simulink model "ForceControl_Quadruped_vmc"  (R2018b)
settings: Solver=FixedStepAuto  StartTime=0.0  StopTime=2  FixedStep=0.001  RelTol=1e-3  EnableMultiTasking=on
undefined symbols (not defined in the file or in its folder): robot, X, Y, Z
libraries: sm_lib x43, nesl_utility x32, Contact_Forces_Lib x4
(part 3 of 3)

== matlab function ForceControl_Quadruped_vmc/controller/inverse kinematics3 ==
  data: x input; y input; z input; shoulder output; hip output; knee output
function [shoulder,hip,knee]= coord2theta(x,y,z)
% L1=75.0;
% L2=415.0;
% L3=408.0;


% temp = (L1*L1+L2*L2-x*x-z*z)/(2*L1*L2);
% if temp>1
%     temp = 1;
% elseif temp<-1
%     temp=1;
% end
% theta2 = pi-acos(temp);
% 
% temp = (x*x+z*z+L1*L1-L2*L2)/(2*sqrt(x*x+z*z)*L1);
% if temp>1
%     temp = 1;
% elseif temp<-1
%     temp=1;
% end
% if(x>0)
%     theta1 = abs(atan(x/z))-acos(temp);
% elseif(x<0)
%     theta1 = -abs(atan(x/z))-acos(temp);
% else
%     theta1 = -acos(temp);

L1=0;
L2=0.4;
L3=0.4;

shoulder=atan(-y/z);

%髋关节到足端长度的平方
L_H2E_2=x*x+(y-L1*sin(shoulder))*(y-L1*sin(shoulder))+(z+L1*cos(shoulder))*(z+L1*cos(shoulder));
%髋关节到足端长度
L_H2E=sqrt(L_H2E_2);

temp = (L2*L2+L_H2E_2-L3*L3)/(2*L_H2E*L2);
if temp>1
    temp = 1;
elseif temp<-1
    temp = -1;
end
Zeta=acos(temp);
hip=atan(x/(sqrt(y*y+z*z)-L1))-Zeta;

temp = (L2*L2+L3*L3-L_H2E_2)/(2*L2*L3);
if temp>1
    temp = 1;
elseif temp<-1
    temp = -1;
end
knee=pi-acos(temp);

== matlab function ForceControl_Quadruped_vmc/controller/inverse kinematics4 ==
  data: x input; y input; z input; shoulder output; hip output; knee output
function [shoulder,hip,knee]= coord2theta(x,y,z)
% L1=75.0;
% L2=415.0;
% L3=408.0;


% temp = (L1*L1+L2*L2-x*x-z*z)/(2*L1*L2);
% if temp>1
%     temp = 1;
% elseif temp<-1
%     temp=1;
% end
% theta2 = pi-acos(temp);
% 
% temp = (x*x+z*z+L1*L1-L2*L2)/(2*sqrt(x*x+z*z)*L1);
% if temp>1
%     temp = 1;
% elseif temp<-1
%     temp=1;
% end
% if(x>0)
%     theta1 = abs(atan(x/z))-acos(temp);
% elseif(x<0)
%     theta1 = -abs(atan(x/z))-acos(temp);
% else
%     theta1 = -acos(temp);

L1=0;
L2=0.4;
L3=0.4;

shoulder=atan(-y/z);

%髋关节到足端长度的平方
L_H2E_2=x*x+(y-L1*sin(shoulder))*(y-L1*sin(shoulder))+(z+L1*cos(shoulder))*(z+L1*cos(shoulder));
%髋关节到足端长度
L_H2E=sqrt(L_H2E_2);

temp = (L2*L2+L_H2E_2-L3*L3)/(2*L_H2E*L2);
if temp>1
    temp = 1;
elseif temp<-1
    temp = -1;
end
Zeta=acos(temp);
hip=atan(x/(sqrt(y*y+z*z)-L1))-Zeta;

temp = (L2*L2+L3*L3-L_H2E_2)/(2*L2*L3);
if temp>1
    temp = 1;
elseif temp<-1
    temp = -1;
end
knee=pi-acos(temp);

== matlab function ForceControl_Quadruped_vmc/controller/trajectory generate1 ==
  data: timer1 input; first_run input; timer1 output; first_run output; LegFL output; LegFR output; LegRR output; LegRL output; run input; roll_angle input; pitch_angle input; yaw_angle input; Body_x input; Body_y input; Body_z input
function [timer1,first_run,LegFL,LegFR,LegRR,LegRL] = gesture( timer1,first_run,run,roll_angle,pitch_angle,yaw_angle,Body_x,Body_y,Body_z)
Ts = 0.75;

if run
    timer1 = timer1+0.001;
    if timer1>=Ts
        timer1 = 0;
    end
end

Xs = -0.1;
Xe = 0.1;

Ys = 0;

Zs = -0.55;
H = 0.15;

body_len_half = 0.35;
body_width_half = 0.2;

Body2FL = [body_len_half,body_width_half,0]';
Body2FR = [body_len_half,-body_width_half,0]';
Body2RR = [-body_len_half,-body_width_half,0]';
Body2RL = [-body_len_half,body_width_half,0]';

Body2FL_trans = [eye(3,3),Body2FL;
    zeros(1,3),1];
Body2FR_trans = [eye(3,3),Body2FR;
    zeros(1,3),1];
Body2RR_trans = [eye(3,3),Body2RR;
    zeros(1,3),1];
Body2RL_trans = [eye(3,3),Body2RL;
    zeros(1,3),1];

roll = roll_angle*pi/180;  
pitch = pitch_angle*pi/180; 
yaw = yaw_angle*pi/180;    

R_roll=[1,0,0,0;
        0,cos(roll),-sin(roll),0;
        0,sin(roll),cos(roll),0;
        0,0,0,1];

R_pitch=[cos(pitch),0,sin(pitch),0;
        0,1,0,0;
        -sin(pitch),0,cos(pitch),0;
        0,0,0,1];

R_yaw=[cos(yaw),-sin(yaw),0,0;
        sin(yaw),cos(yaw),0,0;
        0,0,1,0;
        0,0,0,1];

Body_Trans=[eye(3,3),[Body_x,Body_y,Body_z]';
            zeros(1,3),1];

if first_run
    if timer1>0 && timer1<=0.5*Ts 
        sigma = 2*pi*(timer1)/(0.5*Ts);
        x_f = (Xe-Xs)*((sigma-sin(sigma))/(2*pi))+Xs;  
        x_b = (Xs-Xe)*((sigma-sin(sigma))/(2*pi))+Xe;  
        z_up = H*(1-cos(sigma))/2+Zs;
        
        LegFL = [Xs,-Ys,Zs]';
        LegFR = [x_f,Ys,z_up]';
        LegRR = [Xs,Ys,Zs]';
        LegRL = [x_f,-Ys,z_up]';
    else
        LegFL = [Xs,-Ys,Zs]';
        LegFR = [Xs,Ys,Zs]';
        LegRR = [Xs,Ys,Zs]';
        LegRL = [Xs,-Ys,Zs]';
    end
    if timer1>0.5*Ts
        timer1 = 0;
        first_run = 0;
    end
else
    if timer1>0 && timer1<=0.5*Ts 
        sigma = 2*pi*(timer1)/(0.5*Ts);
        x_f = (Xe-Xs)*((sigma-sin(sigma))/(2*pi))+Xs;  
        x_b = (Xs-Xe)*((sigma-sin(sigma))/(2*pi))+Xe;  
        z_up = H*(1-cos(sigma))/2+Zs; 
        
        O_FL = [body_len_half+x_f,body_width_half,z_up,1]';
        O_FR = [body_len_half+x_b,-body_width_half,Zs,1]';
        O_RR = [-body_len_half+x_f,-body_width_half,z_up,1]';
        O_RL = [-body_len_half+x_b,body_width_half,Zs,1]';
        
    elseif timer1>0.5*Ts && timer1<Ts 
        sigma = 2*pi*(timer1-0.5*Ts)/(0.5*Ts);
        x_f = (Xe-Xs)*((sigma-sin(sigma))/(2*pi))+Xs;
        x_b = (Xs-Xe)*((sigma-sin(sigma))/(2*pi))+Xe;  
        z_up = H*(1-cos(sigma))/2+Zs;
              
        O_FL = [body_len_half+x_b,body_width_half,Zs,1]';
        O_FR = [body_len_half+x_f,-body_width_half,z_up,1]';
        O_RR = [-body_len_half+x_b,-body_width_half,Zs,1]';
        O_RL = [-body_len_half+x_f,body_width_half,z_up,1]';
    else 
        roll = 0;
        pitch = 0;
        yaw = 0;
        Body_x = 0;
        Body_y = 0;
        Body_z = 0;
        
        R_roll=[1,0,0,0;
                0,cos(roll),-sin(roll),0;
                0,sin(roll),cos(roll),0;
                0,0,0,1];
        R_pitch=[cos(pitch),0,sin(pitch),0;
                0,1,0,0;
                -sin(pitch),0,cos(pitch),0;
                0,0,0,1];
        R_yaw=[cos(yaw),-sin(yaw),0,0;
                sin(yaw),cos(yaw),0,0;
                0,0,1,0;
                0,0,0,1];
        Body_Trans=[eye(3,3),[Body_x,Body_y,Body_z]';
                    zeros(1,3),1];
        O_FL = [body_len_half+Xs,body_width_half-Ys,Zs,1]';
        O_FR = [body_len_half+Xs,-body_width_half+Ys,Zs,1]';
        O_RR = [-body_len_half+Xs,-body_width_half+Ys,Zs,1]';
        O_RL = [-body_len_half+Xs,body_width_half-Ys,Zs,1]';
    end
    P_FL = inv(Body2FL_trans)*R_roll*R_pitch*R_yaw*Body_Trans*O_FL;
    P_FR = inv(Body2FR_trans)*R_roll*R_pitch*R_yaw*Body_Trans*O_FR;
    P_RR = inv(Body2RR_trans)*R_roll*R_pitch*R_yaw*Body_Trans*O_RR;
    P_RL = inv(Body2RL_trans)*R_roll*R_pitch*R_yaw*Body_Trans*O_RL;

    LegFL = P_FL(1:3);
    LegFR = P_FR(1:3);
    LegRR = P_RR(1:3);
    LegRL = P_RL(1:3);
end

== matlab function ForceControl_Quadruped_vmc/controller/inverse kinematics2 ==
  data: x input; y input; z input; shoulder output; hip output; knee output
function [shoulder,hip,knee]= coord2theta(x,y,z)
% L1=75.0;
% L2=415.0;
% L3=408.0;


% temp = (L1*L1+L2*L2-x*x-z*z)/(2*L1*L2);
% if temp>1
%     temp = 1;
% elseif temp<-1
%     temp=1;
% end
% theta2 = pi-acos(temp);
% 
% temp = (x*x+z*z+L1*L1-L2*L2)/(2*sqrt(x*x+z*z)*L1);
% if temp>1
%     temp = 1;
% elseif temp<-1
%     temp=1;
% end
% if(x>0)
%     theta1 = abs(atan(x/z))-acos(temp);
% elseif(x<0)
%     theta1 = -abs(atan(x/z))-acos(temp);
% else
%     theta1 = -acos(temp);

L1=0;
L2=0.4;
L3=0.4;

shoulder=atan(-y/z);

%髋关节到足端长度的平方
L_H2E_2=x*x+(y-L1*sin(shoulder))*(y-L1*sin(shoulder))+(z+L1*cos(shoulder))*(z+L1*cos(shoulder));
%髋关节到足端长度
L_H2E=sqrt(L_H2E_2);

temp = (L2*L2+L_H2E_2-L3*L3)/(2*L_H2E*L2);
if temp>1
    temp = 1;
elseif temp<-1
    temp = -1;
end
Zeta=acos(temp);
hip=atan(x/(sqrt(y*y+z*z)-L1))-Zeta;

temp = (L2*L2+L3*L3-L_H2E_2)/(2*L2*L3);
if temp>1
    temp = 1;
elseif temp<-1
    temp = -1;
end
knee=pi-acos(temp);

== matlab function ForceControl_Quadruped_vmc/FL/MATLAB Function1 ==
  data: q input; coord output
function coord = forward_kinematics(q)

%肩关节中心为坐标原点
%坐标轴满足右手定则，x轴朝右，z轴朝上，逆时针为旋转正方向

%L0(shoulder length) L1(upper leg length) L2(lower leg length)
%theta0(shoulder angle) theta1(hip angle) theta2(knee angle)

%     x = L1*sin(theta1)+L2*sin(theta1+theta2);
%     y = sin(theta0)*(L1*cos(theta1)+L2*cos(theta1+theta2));
%     z = -cos(theta0)*(L1*cos(theta1)+L2*cos(theta1+theta2));

theta0 = q(1);
theta1 = q(2);
theta2 = q(3);

L0 = 0;
L1 = 0.4;
L2 = 0.4;

s0 = sin(theta0);s1 = sin(theta1);s2 = sin(theta2);
c0 = cos(theta0);c1 = cos(theta1);c2 = cos(theta2);
s12 = sin(theta1+theta2);c12 = cos(theta1+theta2);

x = L1*s1+L2*s12;
y = s0*(L1*c1+L2*c12);
z = -c0*(L1*c1+L2*c12);

coord = [x,y,z];

== matlab function ForceControl_Quadruped_vmc/FL/MATLAB Function2 ==
  data: pos input; vel output; pos_last input; pos output; first_run input; first_run output
function [vel,pos,first_run] = Pos2Vel(pos,pos_last,first_run)

if first_run
    x_pos_last = pos(1);
    y_pos_last = pos(2);
    z_pos_last = pos(3);
    first_run = 0;
else
    x_pos_last = pos_last(1);
    y_pos_last = pos_last(2);
    z_pos_last = pos_last(3);
end

x_pos = pos(1);
y_pos = pos(2);
z_pos = pos(3);

x_vel = (x_pos-x_pos_last)/0.001;
y_vel = (y_pos-y_pos_last)/0.001;
z_vel = (z_pos-z_pos_last)/0.001;

vel = [x_vel,y_vel,z_vel];

== matlab function ForceControl_Quadruped_vmc/FL/MATLAB Function ==
  data: fx input; tau0 output; fy input; fz input; tau1 output; tau2 output; theta input
function [tau0,tau1,tau2] = fcn(fx,fy,fz,theta)
L0 = 0;
L1 = 0.4;
L2 = 0.4;

theta0 = theta(1);theta1 = theta(2);theta2 = theta(3);
s0 = sin(theta0);s1 = sin(theta1);s2 = sin(theta2);
c0 = cos(theta0);c1 = cos(theta1);c2 = cos(theta2);
s12 = sin(theta1+theta2);c12 = cos(theta1+theta2);

% x = L1*s1+L2*s12;
% y = s0*(L1*c1+L2*c12);
% z = -c0*(L1*c1+L2*c12);


J = [0 L1*c1+L2*c12 L2*c12;
    c0*(L1*c1+L2*c12) -s0*(L1*s1+L2*s12) -s0*(L2*s12);
    s0*(L1*c1+L2*c12) c0*(L1*s1+L2*s12) c0*(L2*s12)];

F = [fx;fy;fz];
tau = J'*F;

tau0 = tau(1);
tau1 = tau(2);
tau2 = tau(3);

== matlab function ForceControl_Quadruped_vmc/FL1/MATLAB Function ==
  data: fx input; tau0 output; fy input; fz input; tau1 output; tau2 output; theta input
function [tau0,tau1,tau2] = fcn(fx,fy,fz,theta)
L0 = 0;
L1 = 0.4;
L2 = 0.4;

theta0 = theta(1);theta1 = theta(2);theta2 = theta(3);
s0 = sin(theta0);s1 = sin(theta1);s2 = sin(theta2);
c0 = cos(theta0);c1 = cos(theta1);c2 = cos(theta2);
s12 = sin(theta1+theta2);c12 = cos(theta1+theta2);

% x = L1*s1+L2*s12;
% y = s0*(L1*c1+L2*c12);
% z = -c0*(L1*c1+L2*c12);


J = [0 L1*c1+L2*c12 L2*c12;
    c0*(L1*c1+L2*c12) -s0*(L1*s1+L2*s12) -s0*(L2*s12);
    s0*(L1*c1+L2*c12) c0*(L1*s1+L2*s12) c0*(L2*s12)];

F = [fx;fy;fz];
tau = J'*F;

tau0 = tau(1);
tau1 = tau(2);
tau2 = tau(3);

== matlab function ForceControl_Quadruped_vmc/FL1/MATLAB Function1 ==
  data: q input; coord output
function coord = forward_kinematics(q)

%肩关节中心为坐标原点
%坐标轴满足右手定则，x轴朝右，z轴朝上，逆时针为旋转正方向

%L0(shoulder length) L1(upper leg length) L2(lower leg length)
%theta0(shoulder angle) theta1(hip angle) theta2(knee angle)

%     x = L1*sin(theta1)+L2*sin(theta1+theta2);
%     y = sin(theta0)*(L1*cos(theta1)+L2*cos(theta1+theta2));
%     z = -cos(theta0)*(L1*cos(theta1)+L2*cos(theta1+theta2));

theta0 = q(1);
theta1 = q(2);
theta2 = q(3);

L0 = 0;
L1 = 0.4;
L2 = 0.4;

s0 = sin(theta0);s1 = sin(theta1);s2 = sin(theta2);
c0 = cos(theta0);c1 = cos(theta1);c2 = cos(theta2);
s12 = sin(theta1+theta2);c12 = cos(theta1+theta2);

x = L1*s1+L2*s12;
y = s0*(L1*c1+L2*c12);
z = -c0*(L1*c1+L2*c12);

coord = [x,y,z];

== matlab function ForceControl_Quadruped_vmc/FL1/MATLAB Function2 ==
  data: pos input; vel output; pos_last input; pos output; first_run input; first_run output
function [vel,pos,first_run] = Pos2Vel(pos,pos_last,first_run)

if first_run
    x_pos_last = pos(1);
    y_pos_last = pos(2);
    z_pos_last = pos(3);
    first_run = 0;
else
    x_pos_last = pos_last(1);
    y_pos_last = pos_last(2);
    z_pos_last = pos_last(3);
end

x_pos = pos(1);
y_pos = pos(2);
z_pos = pos(3);

x_vel = (x_pos-x_pos_last)/0.001;
y_vel = (y_pos-y_pos_last)/0.001;
z_vel = (z_pos-z_pos_last)/0.001;

vel = [x_vel,y_vel,z_vel];

== matlab function ForceControl_Quadruped_vmc/FL2/MATLAB Function ==
  data: fx input; tau0 output; fy input; fz input; tau1 output; tau2 output; theta input
function [tau0,tau1,tau2] = fcn(fx,fy,fz,theta)
L0 = 0;
L1 = 0.4;
L2 = 0.4;

theta0 = theta(1);theta1 = theta(2);theta2 = theta(3);
s0 = sin(theta0);s1 = sin(theta1);s2 = sin(theta2);
c0 = cos(theta0);c1 = cos(theta1);c2 = cos(theta2);
s12 = sin(theta1+theta2);c12 = cos(theta1+theta2);

% x = L1*s1+L2*s12;
% y = s0*(L1*c1+L2*c12);
% z = -c0*(L1*c1+L2*c12);


J = [0 L1*c1+L2*c12 L2*c12;
    c0*(L1*c1+L2*c12) -s0*(L1*s1+L2*s12) -s0*(L2*s12);
    s0*(L1*c1+L2*c12) c0*(L1*s1+L2*s12) c0*(L2*s12)];

F = [fx;fy;fz];
tau = J'*F;

tau0 = tau(1);
tau1 = tau(2);
tau2 = tau(3);

== matlab function ForceControl_Quadruped_vmc/FL2/MATLAB Function1 ==
  data: q input; coord output
function coord = forward_kinematics(q)

%肩关节中心为坐标原点
%坐标轴满足右手定则，x轴朝右，z轴朝上，逆时针为旋转正方向

%L0(shoulder length) L1(upper leg length) L2(lower leg length)
%theta0(shoulder angle) theta1(hip angle) theta2(knee angle)

%     x = L1*sin(theta1)+L2*sin(theta1+theta2);
%     y = sin(theta0)*(L1*cos(theta1)+L2*cos(theta1+theta2));
%     z = -cos(theta0)*(L1*cos(theta1)+L2*cos(theta1+theta2));

theta0 = q(1);
theta1 = q(2);
theta2 = q(3);

L0 = 0;
L1 = 0.4;
L2 = 0.4;

s0 = sin(theta0);s1 = sin(theta1);s2 = sin(theta2);
c0 = cos(theta0);c1 = cos(theta1);c2 = cos(theta2);
s12 = sin(theta1+theta2);c12 = cos(theta1+theta2);

x = L1*s1+L2*s12;
y = s0*(L1*c1+L2*c12);
z = -c0*(L1*c1+L2*c12);

coord = [x,y,z];

== matlab function ForceControl_Quadruped_vmc/FL2/MATLAB Function2 ==
  data: pos input; vel output; pos_last input; pos output; first_run input; first_run output
function [vel,pos,first_run] = Pos2Vel(pos,pos_last,first_run)

if first_run
    x_pos_last = pos(1);
    y_pos_last = pos(2);
    z_pos_last = pos(3);
    first_run = 0;
else
    x_pos_last = pos_last(1);
    y_pos_last = pos_last(2);
    z_pos_last = pos_last(3);
end

x_pos = pos(1);
y_pos = pos(2);
z_pos = pos(3);

x_vel = (x_pos-x_pos_last)/0.001;
y_vel = (y_pos-y_pos_last)/0.001;
z_vel = (z_pos-z_pos_last)/0.001;

vel = [x_vel,y_vel,z_vel];

== matlab function ForceControl_Quadruped_vmc/FL3/MATLAB Function ==
  data: fx input; tau0 output; fy input; fz input; tau1 output; tau2 output; theta input
function [tau0,tau1,tau2] = fcn(fx,fy,fz,theta)
L0 = 0;
L1 = 0.4;
L2 = 0.4;

theta0 = theta(1);theta1 = theta(2);theta2 = theta(3);
s0 = sin(theta0);s1 = sin(theta1);s2 = sin(theta2);
c0 = cos(theta0);c1 = cos(theta1);c2 = cos(theta2);
s12 = sin(theta1+theta2);c12 = cos(theta1+theta2);

% x = L1*s1+L2*s12;
% y = s0*(L1*c1+L2*c12);
% z = -c0*(L1*c1+L2*c12);


J = [0 L1*c1+L2*c12 L2*c12;
    c0*(L1*c1+L2*c12) -s0*(L1*s1+L2*s12) -s0*(L2*s12);
    s0*(L1*c1+L2*c12) c0*(L1*s1+L2*s12) c0*(L2*s12)];

F = [fx;fy;fz];
tau = J'*F;

tau0 = tau(1);
tau1 = tau(2);
tau2 = tau(3);

== matlab function ForceControl_Quadruped_vmc/FL3/MATLAB Function1 ==
  data: q input; coord output
function coord = forward_kinematics(q)

%肩关节中心为坐标原点
%坐标轴满足右手定则，x轴朝右，z轴朝上，逆时针为旋转正方向

%L0(shoulder length) L1(upper leg length) L2(lower leg length)
%theta0(shoulder angle) theta1(hip angle) theta2(knee angle)

%     x = L1*sin(theta1)+L2*sin(theta1+theta2);
%     y = sin(theta0)*(L1*cos(theta1)+L2*cos(theta1+theta2));
%     z = -cos(theta0)*(L1*cos(theta1)+L2*cos(theta1+theta2));

theta0 = q(1);
theta1 = q(2);
theta2 = q(3);

L0 = 0;
L1 = 0.4;
L2 = 0.4;

s0 = sin(theta0);s1 = sin(theta1);s2 = sin(theta2);
c0 = cos(theta0);c1 = cos(theta1);c2 = cos(theta2);
s12 = sin(theta1+theta2);c12 = cos(theta1+theta2);

x = L1*s1+L2*s12;
y = s0*(L1*c1+L2*c12);
z = -c0*(L1*c1+L2*c12);

coord = [x,y,z];

== matlab function ForceControl_Quadruped_vmc/FL3/MATLAB Function2 ==
  data: pos input; vel output; pos_last input; pos output; first_run input; first_run output
function [vel,pos,first_run] = Pos2Vel(pos,pos_last,first_run)

if first_run
    x_pos_last = pos(1);
    y_pos_last = pos(2);
    z_pos_last = pos(3);
    first_run = 0;
else
    x_pos_last = pos_last(1);
    y_pos_last = pos_last(2);
    z_pos_last = pos_last(3);
end

x_pos = pos(1);
y_pos = pos(2);
z_pos = pos(3);

x_vel = (x_pos-x_pos_last)/0.001;
y_vel = (y_pos-y_pos_last)/0.001;
z_vel = (z_pos-z_pos_last)/0.001;

vel = [x_vel,y_vel,z_vel];

== matlab function ForceControl_Quadruped_vmc/controller1/MATLAB Function ==
  data: t input; theta_t output; theta_t_d output; theta_t_d2 output
function [theta_t,theta_t_d,theta_t_d2] = traj(t)

tf=2;
theta_0=0;
theta_f=pi/6;

a0=theta_0;
a1=0;
a2=3/(tf^2)*(theta_f-theta_0);
a3=-2/(tf^3)*(theta_f-theta_0);

theta_t=a0+a1.*t+a2.*t.^2+a3.*t.^3;
theta_t_d=a1+2*a2.*t+3*a3*t.^2;
theta_t_d2=2*a2+6*a3.*t;

== matlab function ForceControl_Quadruped_vmc/controller1/MATLAB Function1 ==
  data: theta input; theta_d input; q input; tau output; q_d input; q_d2 input
function tau  = dynamics(theta,theta_d,q,q_d,q_d2)
%DYNAMICS 此处显示有关此函数的摘要
%   此处显示详细说明
% I=1/12*m*(L1^2+L2^2) 
% 质量50KG，长宽高分别为0.8，0.4，0.2
% x轴，y轴，z轴分别平行于长宽高方向，原点建立在几何中心
mp = 50;

Ix=1/12*mp*(0.4^2+0.2^2);
Iy=1/12*mp*(0.8^2+0.2^2);
Iz=1/12*mp*(0.8^2+0.4^2);

theta_x=theta(1);theta_y=theta(2);theta_z=theta(3);
theta_x_d=theta_d(1);theta_y_d=theta_d(2);theta_z_d=theta_d(3);

sx=sin(theta_x);sy=sin(theta_y);sz=sin(theta_z);
cx=cos(theta_x);cy=cos(theta_y);cz=cos(theta_z);

m11=mp; m22=mp; m33=mp; m44=Ix*cy^2*cz^2+Iy*cy^2*sz^2+Iz*sy^2;
m45=(Ix-Iy)*cy*sz*cz; m46=Iz*sy; m54=(Ix-Iy)*cy*sz*cz;
m55=Ix*sz^2+Iy*cz^2; m64=Iz*sy; m66=Iz;

M = [m11,0,0,0,0,0;
     0,m22,0,0,0,0;
     0,0,m33,0,0,0;
     0,0,0,m44,m45,m46;
     0,0,0,m54,m55,0;
     0,0,0,m64,0,m66;];
 
 k1=-cy*sy*(cz^2*Ix+sz^2*Iy-Iz); k2=-cy^2*cz*sz*(Ix-Iy);
 k3=(cz-sz)*(cz+sz)*(Ix-Iy)*cy/2; k4=cz*sz*(Ix-Iy);
 k5=-cz*sz*sy*(Ix-Iy); k6=Iz*cy/2;
 
 c44=k1*theta_y_d+k2*theta_z_d; 
 c45=k1*theta_x_d+k5*theta_y_d+(k3+k6)*theta_z_d;
 c46=k2*theta_x_d+(k3+k6)*theta_y_d;
 c54=-k1*theta_x_d+(k3-k6)*theta_z_d;
 c55=k4*theta_z_d;
 c56=k4*theta_y_d+(k3-k6)*theta_x_d;
 c64=-k2*theta_x_d+(k6-k3)*theta_y_d;
 c65=(k6-k3)*theta_x_d-k4*theta_y_d;
 
 C=[zeros(3,6);
     0,0,0,c44,c45,c46;
     0,0,0,c54,c55,c56;
     0,0,0,c64,c65,0];
 
 G=[0,0,mp*9.81,0,0,0]';
 
 tau=M*q_d2+C*q_d+G;
 
end

== matlab function ForceControl_Quadruped_vmc/body/MATLAB Function3 ==
  data: q input; roll output; pitch output; yaw output
function [roll,pitch,yaw] = quaternion2eular(q)

qw=q(1);qx=q(2);qy=q(3);qz=q(4);

roll=atan2(2*(qw*qx+qy*qz),1-2*(qx^2+qy^2));
pitch=asin(2*(qw*qy-qz*qx));
yaw=atan2(2*(qw*qz+qx*qy),1-2*(qy^2+qz^2));

== matlab function ForceControl_Quadruped_vmc/controller1/MATLAB Function4 ==
  data: theta input; J output
function J = jacobian(theta)


roll=theta(1);
pitch=theta(2);
yaw=theta(3);

P1=[0.4;0.2;0];P2=[0.4;-0.2;0];P3=[-0.4;-0.2;0];P4=[-0.4;0.2;0];

Ax=[1,0,0;
    0,cos(roll),-sin(roll);
    0,sin(roll),cos(roll);];

Ay=[cos(pitch),0,sin(pitch);
    0,1,0;
    -sin(pitch),0,cos(pitch);];

Az=[cos(yaw),-sin(yaw),0;
    sin(yaw),cos(yaw),0;
    0,0,1;];

Si=[0,0,0;
    0,0,-1;
    0,1,0;];
Sj=[0,0,1;
    0,0,0;
    -1,0,0;];
Sk=[0,-1,0;
    1,0,0;
    0,0,0;];

J = [eye(3,3),Az*Ay*Si*Ax*P1,Az*Sj*Ay*Ax*P1,Sk*Az*Ay*Ax*P1;
    eye(3,3),Az*Ay*Si*Ax*P2,Az*Sj*Ay*Ax*P2,Sk*Az*Ay*Ax*P2;
    eye(3,3),Az*Ay*Si*Ax*P3,Az*Sj*Ay*Ax*P3,Sk*Az*Ay*Ax*P3;
    eye(3,3),Az*Ay*Si*Ax*P4,Az*Sj*Ay*Ax*P4,Sk*Az*Ay*Ax*P4;];
J = pinv(J');
